simulink model "gain_test_Kuuvect"  (Simulink 9.0)
settings: Solver=FixedStepAuto  StartTime=0.0  StopTime=10.0  FixedStep=0.1  RelTol=1e-3  EnableMultiTasking=on
settings Model: SuppressorTable=22 serialization::archive 11 0 6 0 0 0 0 0  Creator=arnaud  LastModifiedBy=hbourbou
settings DataIOCC: LimitDataPoints=on  SaveFormat=Structure  SignalLoggingSaveFormat=ModelDataLogs
settings OptimizationCC: ExpressionDepthLimit=2147483647
settings DebuggingCC: SolverPrmCheckMsg=warning  FcnCallInpInsideContextMsg=warning  StateNameClashWarn=warning  StrictBusMsg=Warning
settings GRTTargetCC: CombineOutputUpdateFcns=off  GRTInterface=on

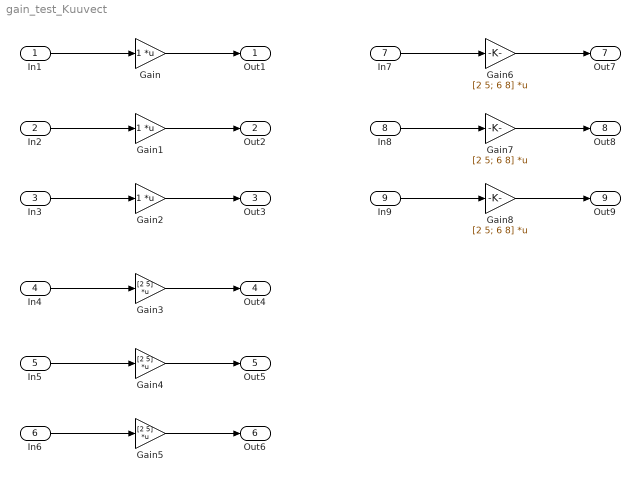
== system gain_test_Kuuvect ==
  In1 : Inport  OutDataTypeStr=double
  In2 : Inport  Port=2  OutDataTypeStr=int8  PortDimensions=1
  In3 : Inport  Port=3  OutDataTypeStr=boolean  PortDimensions=1
  In4 : Inport  Port=4  OutDataTypeStr=double  PortDimensions=2
  In5 : Inport  Port=5  OutDataTypeStr=int8  PortDimensions=2
  In6 : Inport  Port=6  OutDataTypeStr=boolean  PortDimensions=2
  In7 : Inport  Port=7  OutDataTypeStr=double  PortDimensions=[2 1]
  In8 : Inport  Port=8  OutDataTypeStr=int8  PortDimensions=2
  In9 : Inport  Port=9  OutDataTypeStr=boolean  PortDimensions=[2 1]
  Gain : Gain  Multiplication=Matrix(K*u) (u vector)
  Gain1 : Gain  Multiplication=Matrix(K*u) (u vector)
  Gain2 : Gain  Multiplication=Matrix(K*u) (u vector)
  Gain3 : Gain  Gain=[2 5]  Multiplication=Matrix(K*u) (u vector)
  Gain4 : Gain  Gain=[2 5]  Multiplication=Matrix(K*u) (u vector)
  Gain5 : Gain  Gain=[2 5]  Multiplication=Matrix(K*u) (u vector)
  Gain6 : Gain  Gain=[2 5; 6 8]  Multiplication=Matrix(K*u) (u vector)
  Gain7 : Gain  Gain=[2 5; 6 8]  Multiplication=Matrix(K*u) (u vector)
  Gain8 : Gain  Gain=[2 5; 6 8]  Multiplication=Matrix(K*u) (u vector)
  Out1 : Outport
  Out2 : Outport  Port=2
  Out3 : Outport  Port=3
  Out4 : Outport  Port=4
  Out5 : Outport  Port=5
  Out6 : Outport  Port=6
  Out7 : Outport  Port=7
  Out8 : Outport  Port=8
  Out9 : Outport  Port=9
  wires:
  In1/1 -> Gain/1
  Gain/1 -> Out1/1
  In2/1 -> Gain1/1
  Gain1/1 -> Out2/1
  In3/1 -> Gain2/1
  Gain2/1 -> Out3/1
  In4/1 -> Gain3/1
  Gain3/1 -> Out4/1
  In5/1 -> Gain4/1
  Gain4/1 -> Out5/1
  In6/1 -> Gain5/1
  Gain5/1 -> Out6/1
  In7/1 -> Gain6/1
  Gain6/1 -> Out7/1
  In8/1 -> Gain7/1
  Gain7/1 -> Out8/1
  In9/1 -> Gain8/1
  Gain8/1 -> Out9/1
